simulink model "Lab6"  (R2024b)
settings: Solver=VariableStepAuto  StartTime=0.0  StopTime=10.0  RelTol=1e-3
settings Model: Creator=usama  LastModifiedBy=usama

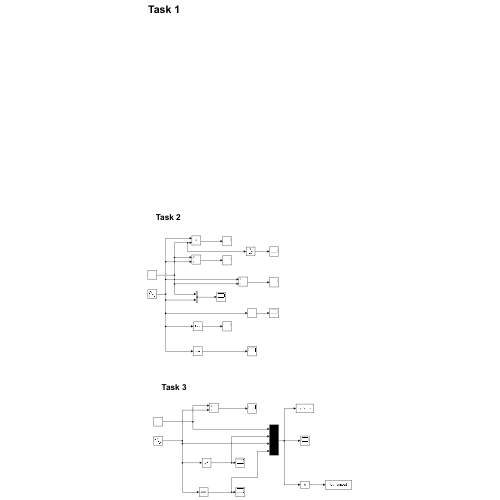
[thumbnail: Simulink's stored preview of the top-level diagram]
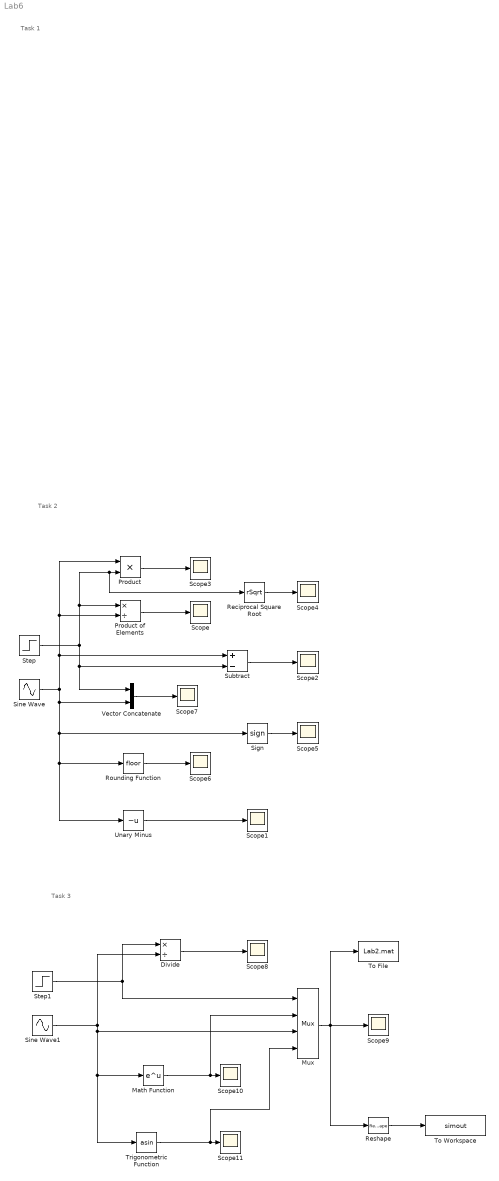
== system Lab6 ==
  note: Task 3
  note: Task 1
  note: Task 2
  Divide : Product  Inputs=*/
  Math Function : Math
  Mux : Mux
  Product : Product
  Product of Elements : Product  Inputs=*/
  Reciprocal Square Root : Sqrt  Operator=rSqrt
  Reshape : Reshape  OutputDimensionality=Customize  OutputDimensions=[2,2]
  Rounding Function : Rounding
  Scope{,1..11} (12 alike) : Scope
  Sign : Signum
  Sine Wave : Sin  SampleTime=0
  Sine Wave1 : Sin  SampleTime=0
  Step : Step  Time=5  SampleTime=0
  Step1 : Step  Time=5  SampleTime=0
  Subtract : Sum  Inputs=+-
  To File : ToFile  Filename=Lab2.mat  SaveFormat=Timeseries
  To Workspace : ToWorkspace  VariableName=simout  SaveFormat=Timeseries  SampleTime=-1
  Trigonometric Function : Trigonometry  Operator=asin
  Unary Minus : UnaryMinus
  Vector Concatenate : Concatenate
  wires:
  Step/1 -> Vector Concatenate/1, Subtract/2, Product of Elements/1, Reciprocal Square Root/1, Product/2
  Product/1 -> Scope3/1
  Sine Wave/1 -> Vector Concatenate/2, Unary Minus/1, Rounding Function/1, Sign/1, Subtract/1, Product of Elements/2, Product/1
  Sign/1 -> Scope5/1
  Unary Minus/1 -> Scope1/1
  Rounding Function/1 -> Scope6/1
  Vector Concatenate/1 -> Scope7/1
  Product of Elements/1 -> Scope/1
  Reciprocal Square Root/1 -> Scope4/1
  Subtract/1 -> Scope2/1
  Step1/1 -> Mux/1, Divide/1
  Sine Wave1/1 -> Mux/3, Trigonometric Function/1, Math Function/1, Divide/2
  Trigonometric Function/1 -> Mux/4, Scope11/1
  Math Function/1 -> Mux/2, Scope10/1
  Mux/1 -> To File/1, Reshape/1, Scope9/1
  Divide/1 -> Scope8/1
  Reshape/1 -> To Workspace/1
